simulink subsystem "Throttle_Map"  (R2023b)
settings: Solver=VariableStepAuto  StartTime=0.0  StopTime=10.0  RelTol=1e-3
undefined symbols (not defined in the file): k_grid_max, k_grid_min, rpm_sweep_min, voltage_sweep_min
settings Model: Creator=Inver  LastModifiedBy=Inver

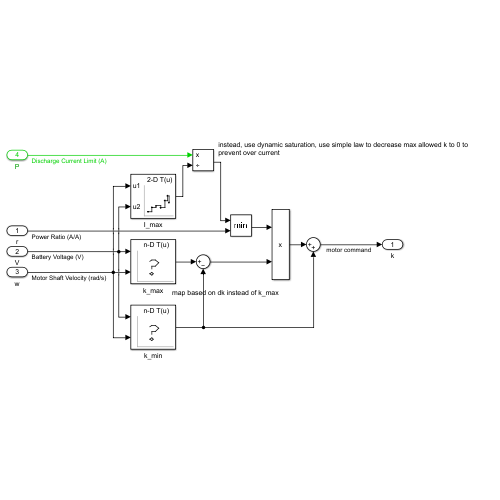
[thumbnail: Simulink's stored preview of the top-level diagram]
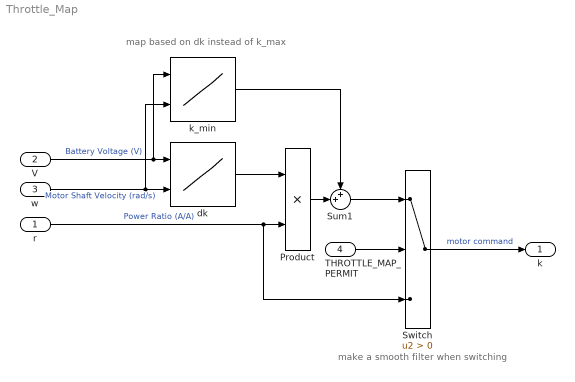
== system Throttle_Map ==
  note: map based on dk instead of k_max
  note: make a smooth filter when switching
  r : Inport
  V : Inport  Port=2
  w : Inport  Port=3
  THROTTLE_MAP_PERMIT : Inport  Port=4
  Product : Product
  Sum1 : Sum  Inputs=++|
  Switch : Switch  Criteria=u2 > Threshold  SaturateOnIntegerOverflow=off  InputSameDT=off
  dk : Lookup_n-D  LookupTableObject=''  BreakpointsForDimension1=voltage_sweep_min  BreakpointsForDimension2=rpm_sweep_min  BreakpointsForDimension1FirstPoint=10  BreakpointsForDimension2FirstPoint=10  BreakpointsForDimension1Spacing=12  BreakpointsForDimension2Spacing=12  IndexSearchMethod=Evenly spaced points  Table=k_grid_max  ExtrapMethod=Clip  DiagnosticForOutOfRangeInput=Error  InternalRulePriority=Speed  RndMeth=Simplest
      settings: InputPortMap=u0,u1
  k_min : Lookup_n-D  LookupTableObject=''  BreakpointsForDimension1=voltage_sweep_min  BreakpointsForDimension2=rpm_sweep_min  BreakpointsForDimension1FirstPoint=10  BreakpointsForDimension2FirstPoint=10  BreakpointsForDimension1Spacing=12  BreakpointsForDimension2Spacing=12  IndexSearchMethod=Evenly spaced points  Table=k_grid_min  ExtrapMethod=Clip  DiagnosticForOutOfRangeInput=Error  InternalRulePriority=Speed  RndMeth=Simplest
      settings: InputPortMap=u0,u1
  k : Outport
  wires:
  w/1 -> k_min/2, dk/2  "Motor Shaft Velocity (rad/s)"
  Switch/1 -> k/1  "motor command"
  V/1 -> k_min/1, dk/1  "Battery Voltage (V)"
  r/1 -> Switch/3, Product/2  "Power Ratio (A/A)"
  THROTTLE_MAP_PERMIT/1 -> Switch/2
  Sum1/1 -> Switch/1
  k_min/1 -> Sum1/1
  Product/1 -> Sum1/2
  dk/1 -> Product/1
